simulink model "PD_g_compen"  (Simulink 7.9)
settings: Solver=ode45  StartTime=0.0  StopTime=10.0  RelTol=1e-3
undefined symbols (not defined in the file): kd1, kd2, kd3, kd4, kd5, kd6, kp1, kp2, kp3, kp4, kp5, kp6, LinePTs2Rpm, PosSourceSelect, Ts
libraries: powerlib_extras x1
settings Model: Creator=Administrator  LastModifiedBy=Administrator

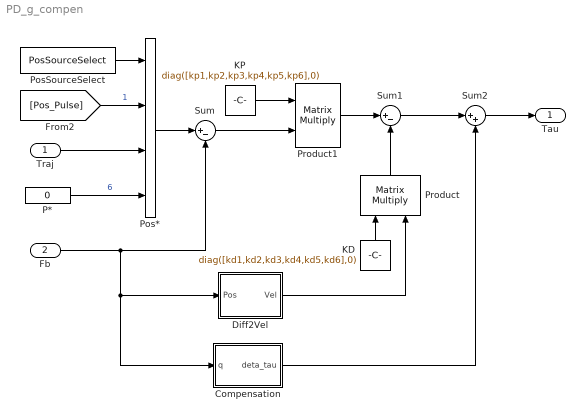
== system PD_g_compen ==
  Traj : Inport
  Fb : Inport  Port=2
  Compensation : Subsystem
  Diff2Vel : Subsystem
  KD : Constant  Value=diag([kd1,kd2,kd3,kd4,kd5,kd6],0)
  KP : Constant  Value=diag([kp1,kp2,kp3,kp4,kp5,kp6],0)
  P* : Constant  Value=0  SampleTime=Ts
  Pos* : MultiPortSwitch  zeroidx=off  SampleTime=Ts
  PosSourceSelect : Constant  Value=PosSourceSelect  SampleTime=Ts
  Product : Product  Multiplication=Matrix(*)  RndMeth=Zero
  Product1 : Product  Multiplication=Matrix(*)  RndMeth=Zero
  Sum : Sum  Inputs=|+-  SampleTime=Ts
  Sum1 : Sum  Inputs=|+-  SampleTime=Ts
  Sum2 : Sum  Inputs=|++  SampleTime=Ts
  Tau : Outport
  wires:
  [Pos_Pulse] -> Pos*/2  "1"
  P*/1 -> Pos*/4  "6"
  PosSourceSelect/1 -> Pos*/1
  Traj/1 -> Pos*/3
  Fb/1 -> Sum/2, Diff2Vel/1(Pos), Compensation/1(q)
  Pos*/1 -> Sum/1
  Product/1 -> Sum1/2
  Sum1/1 -> Sum2/1
  Compensation/1(deta_tau) -> Sum2/2
  Sum2/1 -> Tau/1
  Diff2Vel/1(Vel) -> Product/2
  KD/1 -> Product/1
  Sum/1 -> Product1/2
  Product1/1 -> Sum1/1
  KP/1 -> Product1/1

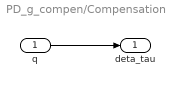
== system PD_g_compen/Compensation ==
  q : Inport
  deta_tau : Outport
  wires:
  q/1 -> deta_tau/1

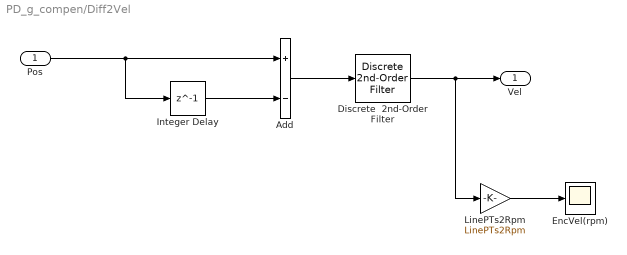
== system PD_g_compen/Diff2Vel ==
  Pos : Inport
  Add : Sum  Inputs=+-
  Discrete  2nd-Order Filter : powerlib_extras/Discrete  Control Blocks/Discrete  2nd-Order Filter  FilterType=Lowpass  Fo=200  Zeta=0.707  Ts=Ts  Initialize=off  Vac_Init=[0.8 -25 60]  Vdc_Init=-0.4  PlotResponse=off  param1=[1 5000 10]
  EncVel(rpm) : Scope
      settings: SaveName=ScopeData33
  Integer Delay : Delay  DelayLength=1  InputProcessing=Inherited
  LinePTs2Rpm : Gain  Gain=LinePTs2Rpm
  Vel : Outport
  wires:
  Add/1 -> Discrete  2nd-Order Filter/1
  Discrete  2nd-Order Filter/1 -> Vel/1, LinePTs2Rpm/1
  Pos/1 -> Integer Delay/1, Add/1
  Integer Delay/1 -> Add/2
  LinePTs2Rpm/1 -> EncVel(rpm)/1
